simulink library "HybridFEMLibrary"  (Simulink 7.0)
undefined symbols (not defined in the file or in its folder): Alpham, DiscIntNeverNeededParam, Elements, gamma1, gamma2, Integrator, Interpolations, sample, SampleRate
(part 2 of 2)

== matlab function Generate Type 1 Element Restoring Force Element/Type 1 Element RF ==
  data: TotalRF output inherited; Element input inherited; Displacement input inherited; NumFreeDOF parameter inherited
% get restoring force for the element
% returns (6x1) restoring force vector of element in global coordinates
function TotalRF  = eml(Element, Displacement, NumFreeDOF)

%% Input mapping
Node1Xcoord = Element(1);
Node1Ycoord = Element(2);
Node2Xcoord = Element(3);
Node2Ycoord = Element(4);
MaterialE = Element(5);
Area = Element(6);
Inertia = Element(7);
Node1UX = Element(8);
Node1UY = Element(9);
Node1THETA = Element(10);
Node2UX = Element(11);
Node2UY = Element(12);
Node2THETA = Element(13);

% Get distance between nodes
X21 = Node2Xcoord - Node1Xcoord;
Y21 = Node2Ycoord - Node1Ycoord;
EL = sqrt(X21 * X21 + Y21 * Y21);
EAL = MaterialE * Area / EL;
EIZL = MaterialE * Inertia / EL;
%calculation of density (the uniform load is only taken into account)
SEP = zeros(6);
SEP(1, 1) = EAL;
SEP(1, 4) = -EAL;
SEP(4, 4) = EAL;
SEP(2, 2) = 12 * EIZL / EL ^ 2;
SEP(2, 3) = 6 * EIZL / EL;
SEP(2, 5) = -SEP(2, 2);
SEP(2, 6) = SEP(2, 3);
SEP(3, 3) = 4 * EIZL;
SEP(3, 5) = -6 * EIZL / EL;
SEP(3, 6) = 2 * EIZL;
SEP(5, 5) = 12 * EIZL / EL ^ 2;
SEP(5, 6) = -6 * EIZL / EL;
SEP(6, 6) = 4 * EIZL;
for i = 1:6
   for j = i:6
      SEP(j, i) = SEP(i, j);
   end
end
DCOS = zeros(3,3);
DCOS(1, 1) = X21 / EL;
DCOS(1, 2) = Y21 / EL;
DCOS(1, 3) = 0;
DCOS(2, 1) = -DCOS(1, 2);
DCOS(2, 2) = DCOS(1, 1);
DCOS(2, 3) = 0;
DCOS(3, 1) = 0;
DCOS(3, 2) = 0;
DCOS(3, 3) = 1;
ALMBDA = zeros(6);       
for i = 1:2
   IK = 3 * (i - 1);
   for j = 1:3
      for k = 1:3
         ALMBDA(j + IK, k + IK) = DCOS(j, k);
      end
   end
end
SE = SEP * ALMBDA;
SEP = SE;
SE = ALMBDA' * SEP;
%create the displacement Ue (6x1) vector of the element in global coordinates
Ue = zeros(6,1);
dof=zeros(6,1);
dof(1,1)=Node1UX;
dof(2,1)=Node1UY;
dof(3,1)=Node1THETA;
dof(4,1)=Node2UX;
dof(5,1)=Node2UY;
dof(6,1)=Node2THETA;
for i=1:6
    if dof(i,1)<=NumFreeDOF
        Ue(i,1)=Displacement(dof(i,1),1);
    end
end
RF = SE * Ue;  %resisting (6x1) resisting force vector of element in global coordinates

% Form total restoring force vector
TotalRF = zeros(NumFreeDOF, 1);
    
% Get element nodes to assemble in the structure restoring force vector
if Node1UX <= NumFreeDOF
    TotalRF(Node1UX, 1) = RF(1, 1);
end
if Node1UY <= NumFreeDOF
    TotalRF(Node1UY, 1) = RF(2, 1);
end
if Node1THETA <= NumFreeDOF
    TotalRF(Node1THETA, 1) = RF(3, 1);
end
if Node2UX <= NumFreeDOF
    TotalRF(Node2UX, 1) = RF(4, 1);
end
if Node2UY <= NumFreeDOF
    TotalRF(Node2UY, 1) = RF(5, 1);
end
if Node2THETA <= NumFreeDOF
    TotalRF(Node2THETA, 1) = RF(6, 1);
end

== matlab function Generate Type 4 Element Restoring Force Element/Type 4 Element RF ==
  data: TotalRF output inherited; Element input inherited; NumFreeDOF parameter inherited; Displacement input inherited
% get restoring force for the element
% returns (6x1) restoring force vector of element in global coordinates
function TotalRF  = eml(Element, NumFreeDOF, Displacement)

%% Input mapping
K11 = Element(1);
K12 = Element(2);
K21 = Element(3);
K22 = Element(4);
Node1UX = Element(5);
Node1UY = Element(6);
Node1THETA = Element(7);
Node2UX = Element(8);
Node2UY = Element(9);
Node2THETA = Element(10);

% preset arrays
SE = zeros(6,6);
    
SE(1, 1) = K11;
SE(1, 4) = K12;
SE(4, 1) = K21;
SE(4, 4) = K22;

%create the displacement Ue (6x1) vector of the element in global coordinates
Ue = zeros(6, 1);
dof=zeros(6,1);
dof(1,1)=Node1UX;
dof(2,1)=Node1UY;
dof(3,1)=Node1THETA;
dof(4,1)=Node2UX;
dof(5,1)=Node2UY;
dof(6,1)=Node2THETA;
for i=1:6
    if dof(i,1)<=NumFreeDOF
        Ue(i,1)=Displacement(dof(i,1),1);
    end
end
RF = SE * Ue;  %resisting (6x1) resisting force vector of element in global coordinates

% Form total restoring force vector
TotalRF = zeros(NumFreeDOF, 1);
    
% Get element nodes to assemble in the structure restoring force vector
if Node1UX <= NumFreeDOF
    TotalRF(Node1UX, 1) = RF(1, 1);
end
if Node1UY <= NumFreeDOF
    TotalRF(Node1UY, 1) = RF(2, 1);
end
if Node1THETA <= NumFreeDOF
    TotalRF(Node1THETA, 1) = RF(3, 1);
end
if Node2UX <= NumFreeDOF
    TotalRF(Node2UX, 1) = RF(4, 1);
end
if Node2UY <= NumFreeDOF
    TotalRF(Node2UY, 1) = RF(5, 1);
end
if Node2THETA <= NumFreeDOF
    TotalRF(Node2THETA, 1) = RF(6, 1);
end

== matlab function Generate Actuator Command/Generate Actuator Command ==
  data: Element input inherited; Command output inherited; Displacement input inherited
% generate the local actuator command
function Command   = fcn(Element, Displacement)

%% Input mapping
Node1UX = Element(1);
Node2UX = Element(4);

% create displacement command
U1 = Displacement(Node1UX);
U2 = Displacement(Node2UX);
Command = U1 - U2;
